simulink model "eDPWMv20matlab2020a"  (R2020a)
settings: Solver=VariableStepAuto  StartTime=0.0  StopTime=Tsim  MaxStep=MaxStep  RelTol=1e-3
values from neighbouring files (symbols this model uses):
  a = 1    [main.m]
  b = 1    [main.m]
  Default_NH = 1    [main.m]
  Default_NL = 0    [main.m]
  fs = 100e3    (= 100000)    [main.m]
  M = 0.3    [main.m]
  MaxStep = Ts/600    (= 1.66666666667e-08)    [main.m]
  PgnH = 1/20    (= 0.05)    [main.m]
  PgnL = 1/2    (= 0.5)    [main.m]
  Ts = 1/fs    (= 1e-05)    [main.m]
  Tsample = 1/fsample    (= 5e-06)    [main.m]
  Tsim = 8000*Ts    (= 0.08)    [main.m]
libraries: dspsigops x3
settings Model: Creator=pel  LastModifiedBy=Giovanni
settings DebuggingCC: UnconnectedInputMsg=none  UnconnectedOutputMsg=none  UnconnectedLineMsg=none
settings ModelReferenceCC: EnableRefExpFcnMdlSchedulingChecks=off
settings RTWCC: Description=Generic Real-Time Target  RTWVerbose=off

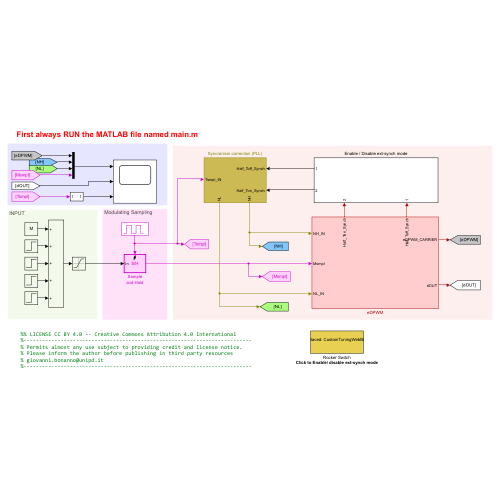
[thumbnail: Simulink's stored preview of the top-level diagram]
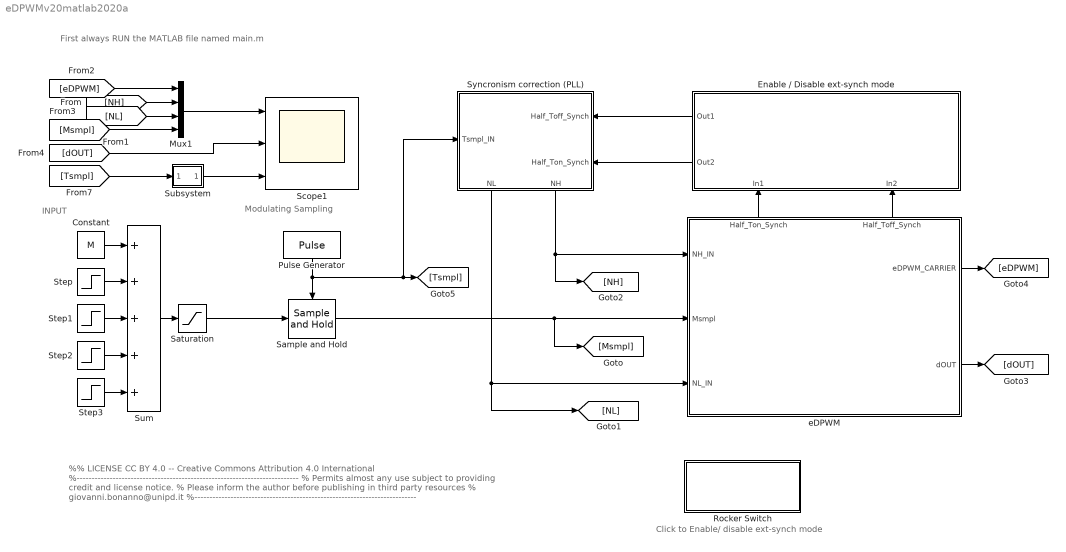
== system eDPWMv20matlab2020a ==
  note: First always RUN the MATLAB file named main.m
  note: Click to Enable/ disable ext-synch mode
  note: %% LICENSE CC BY 4.0 -- Creative Commons Attribution 4.0 International
      | %--------------------------------------------------------------------------
      | % Permits almost any use subject to providing credit and license notice.
      | % Please inform the author before publishing in third party resources
      | % giovanni.bonanno@unipd.it
      | %--------------------------------------------------------------------------
  note: Modulating Sampling
  note: INPUT
  Constant : Constant  Value=M  SampleTime=MaxStep
  Enable / Disable ext-synch mode : Subsystem
      settings: PortSchema="{\"entries\":[{\"content\":{\"sides\":[{\"content\":{},\"type\":\"ConnectorPlacement.EquallySpacedRectSide\",\"uuid\":\"202ee470-7674-402d-b318-20dd7def3ef2\"},{\"content\":{\"connectorIds\":[\"Out1\",\"Out2\"],\"side\":\"RIGHT\"},\"type\":\"ConnectorPlacement.EquallySpacedRectSide\",\"uuid\":\"6d0846ec-2558-4ef4-8253-932ba88cb3e0\"},{\"content\":{\"side\":\"TOP\"},\"type\":\"ConnectorPlacement.EquallySpacedRectSide\",\"uuid\":\"6d21b35b-35b5-4f81-8190-ca95fc47349c\"},{\"content\":{\"connectorIds\":[\"In1\",\"In2\"],\"side\":\"BOTTOM\"},\"type\":\"ConnectorPlacement.EquallySpacedRectSide\",\"uuid\":\"7a5dac1a-5bab-41fb-a369-e6d9d4d78f57\"}]},\"type\":\"ConnectorPlacement.EquallySpacedConnector\",\"uuid\":\"1e7bac81-8cd1-438e-9b37-227f8a4a31bc\"}],\"packageUris\":[\"http://schema.mathworks.com/mf0/Connector/R2020b\"],\"version\":\"1.0\"}"
  Mux1 : Mux
  Pulse Generator : DiscretePulseGenerator  PulseType=Time based  Period=Tsample  PulseWidth=50
  Rocker Switch : Subsystem  Description=Replaced Block  mask(Replaced Block){}
      mask help: This block has been replaced with an empty subsystem because it used functionality that is unavailable in Simulink R2020a.
      mask Display: fprintf('Replaced: %s\n','CustomTuningWebBlock')
  Sample and Hold : dspsigops/Sample and Hold  trig=Rising edge  initCond=M  latchinput=off
  Saturation : Saturate  UpperLimit=1  LowerLimit=0
  Scope1 : Scope  NumInputPorts=3
  Step : Step  Time=Ts*18-Ts/4  After=M/5  SampleTime=MaxStep
  Step1 : Step  Time=Ts*17+Ts/4  After=M/5  SampleTime=MaxStep
  Step2 : Step  Time=Tsim/18+Ts/4+Ts/2  After=M/20  SampleTime=MaxStep
  Step3 : Step  Time=Tsim/18+Ts/4+Ts  After=M/20  SampleTime=MaxStep
  Subsystem : Subsystem
  Sum : Sum  Inputs=+++++
  Syncronism correction (PLL) : Subsystem
      settings: PortSchema="{\"entries\":[{\"content\":{\"sides\":[{\"content\":{\"connectorIds\":[\"In1\"]},\"type\":\"ConnectorPlacement.EquallySpacedRectSide\",\"uuid\":\"af3382a3-5650-4608-9daa-49500a505952\"},{\"content\":{\"connectorIds\":[\"In2\",\"In3\"],\"side\":\"RIGHT\"},\"type\":\"ConnectorPlacement.EquallySpacedRectSide\",\"uuid\":\"51c7e400-8917-4fd6-8211-c90393d7470e\"},{\"content\":{\"side\":\"TOP\"},\"type\":\"ConnectorPlacement.EquallySpacedRectSide\",\"uuid\":\"30f0f9c1-e41e-4d95-bf06-70fe739465e7\"},{\"content\":{\"connectorIds\":[\"Out1\",\"Out2\"],\"side\":\"BOTTOM\"},\"type\":\"ConnectorPlacement.EquallySpacedRectSide\",\"uuid\":\"2c796cb0-67f8-4f41-8e4d-8aa9d4353e04\"}]},\"type\":\"ConnectorPlacement.EquallySpacedConnector\",\"uuid\":\"0b00b238-9597-4f72-adc3-115ce80e6692\"}],\"packageUris\":[\"http://schema.mathworks.com/mf0/Connector/R2020b\"],\"version\":\"1.0\"}"
  eDPWM : Subsystem
      settings: PortSchema="{\"entries\":[{\"content\":{\"sides\":[{\"content\":{\"connectorIds\":[\"In1\",\"In2\",\"In3\"]},\"type\":\"ConnectorPlacement.EquallySpacedRectSide\",\"uuid\":\"bf982af5-63e8-4a41-b560-11889742b778\"},{\"content\":{\"connectorIds\":[\"Out1\",\"Out2\"],\"side\":\"RIGHT\"},\"type\":\"ConnectorPlacement.EquallySpacedRectSide\",\"uuid\":\"a7efdfb9-974d-4c29-9fbc-b41dc0a107af\"},{\"content\":{\"connectorIds\":[\"Out3\",\"Out4\"],\"side\":\"TOP\"},\"type\":\"ConnectorPlacement.EquallySpacedRectSide\",\"uuid\":\"a9c88e29-f7b6-4c63-8087-8b423cce12c8\"},{\"content\":{\"side\":\"BOTTOM\"},\"type\":\"ConnectorPlacement.EquallySpacedRectSide\",\"uuid\":\"491d2149-b1e6-45d2-9cf1-74bcedeaf42d\"}]},\"type\":\"ConnectorPlacement.EquallySpacedConnector\",\"uuid\":\"8fa54b55-faee-4312-8aec-5ed5b37487a1\"}],\"packageUris\":[\"http://schema.mathworks.com/mf0/Connector/R2020b\"],\"version\":\"1.0\"}"
  wires:
  [NH] -> Mux1/2
  [eDPWM] -> Mux1/1
  [Msmpl] -> Mux1/4
  Saturation/1 -> Sample and Hold/1
  [NL] -> Mux1/3
  Mux1/1 -> Scope1/1
  [dOUT] -> Scope1/2
  Sum/1 -> Saturation/1
  Sample and Hold/1 -> eDPWM/2(Msmpl), [Msmpl]
  Pulse Generator/1 -> Sample and Hold/Trigger, Syncronism correction (PLL)/1(Tsmpl_IN), [Tsmpl]
  [Tsmpl] -> Subsystem/1(Inport)
  eDPWM/2(dOUT) -> [dOUT]
  Syncronism correction (PLL)/1(NL) -> eDPWM/3(NL_IN), [NL]
  Syncronism correction (PLL)/2(NH) -> eDPWM/1(NH_IN), [NH]
  eDPWM/1(eDPWM_CARRIER) -> [eDPWM]
  Subsystem/1(Out1) -> Scope1/3
  Constant/1 -> Sum/1
  Step/1 -> Sum/2
  Step1/1 -> Sum/3
  Step2/1 -> Sum/4
  Step3/1 -> Sum/5
  eDPWM/3(Half_Ton_Synch) -> Enable / Disable ext-synch mode/2(In1)
  eDPWM/4(Half_Toff_Synch) -> Enable / Disable ext-synch mode/1(In2)
  Enable / Disable ext-synch mode/1(Out1) -> Syncronism correction (PLL)/2(Half_Toff_Synch)
  Enable / Disable ext-synch mode/2(Out2) -> Syncronism correction (PLL)/3(Half_Ton_Synch)

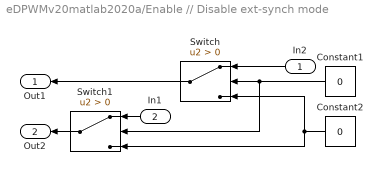
== system eDPWMv20matlab2020a/Enable // Disable ext-synch mode ==
  In2 : Inport
  In1 : Inport  Port=2
  Constant1 : Constant  Value=0
  Constant2 : Constant  Value=0
  Switch : Switch  Criteria=u2 > Threshold
  Switch1 : Switch  Criteria=u2 > Threshold
  Out1 : Outport
  Out2 : Outport  Port=2
  wires:
  In1/1 -> Switch1/1
  Constant2/1 -> Switch1/3, Switch/3
  In2/1 -> Switch/1
  Constant1/1 -> Switch1/2, Switch/2
  Switch1/1 -> Out2/1
  Switch/1 -> Out1/1

== system eDPWMv20matlab2020a/Rocker Switch ==

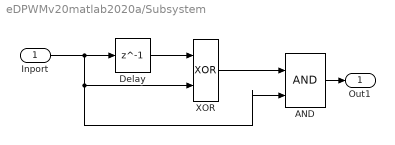
== system eDPWMv20matlab2020a/Subsystem ==
  Inport : Inport
  AND : Logic  IconShape=distinctive  AllPortsSameDT=off  OutDataTypeStr=boolean
  Delay : Delay  DelayLength=1  SampleTime=MaxStep
  XOR : Logic  Operator=XOR  IconShape=distinctive  AllPortsSameDT=off  OutDataTypeStr=boolean
  Out1 : Outport
  wires:
  Inport/1 -> AND/2, XOR/2, Delay/1
  Delay/1 -> XOR/1
  XOR/1 -> AND/1
  AND/1 -> Out1/1

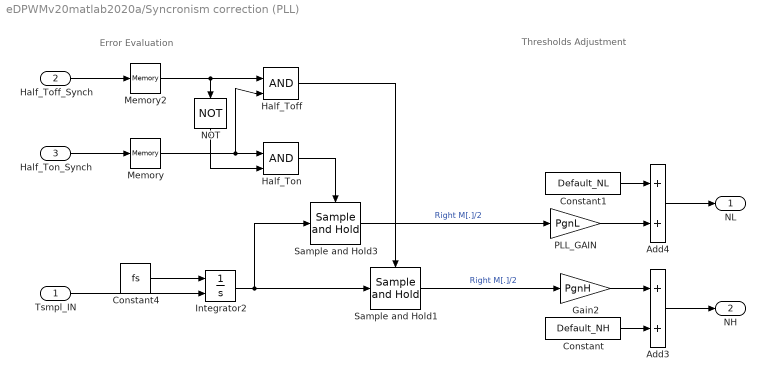
== system eDPWMv20matlab2020a/Syncronism correction (PLL) ==
  note: Thresholds Adjustment
  note: Error Evaluation
  Tsmpl_IN : Inport
  Half_Toff_Synch : Inport  Port=2
  Half_Ton_Synch : Inport  Port=3
  Add3 : Sum
  Add4 : Sum
  Constant : Constant  Value=Default_NH
  Constant1 : Constant  Value=Default_NL
  Constant4 : Constant  Value=fs
  Gain2 : Gain  Gain=PgnH
  Half_Toff : Logic  IconShape=distinctive  AllPortsSameDT=off  OutDataTypeStr=boolean
  Half_Ton : Logic  IconShape=distinctive  AllPortsSameDT=off  OutDataTypeStr=boolean
  Integrator2 : Integrator  ExternalReset=falling  InitialCondition=-0.25  UpperSaturationLimit=0.25  LowerSaturationLimit=-0.25
  Memory : Memory
  Memory2 : Memory
  NOT : Logic  Operator=NOT  IconShape=distinctive  AllPortsSameDT=off  OutDataTypeStr=boolean
  PLL_GAIN : Gain  Gain=PgnL
  Sample and Hold1 : dspsigops/Sample and Hold  trig=Rising edge  initCond=0  latchinput=off
  Sample and Hold3 : dspsigops/Sample and Hold  trig=Rising edge  initCond=0  latchinput=off
  NL : Outport
  NH : Outport  Port=2
  wires:
  Constant4/1 -> Integrator2/1
  Half_Ton/1 -> Sample and Hold3/Trigger
  Tsmpl_IN/1 -> Integrator2/2
  Half_Toff/1 -> Sample and Hold1/Trigger
  NOT/1 -> Half_Ton/2
  Half_Ton_Synch/1 -> Memory/1
  Constant1/1 -> Add4/1
  PLL_GAIN/1 -> Add4/2
  Constant/1 -> Add3/2
  Gain2/1 -> Add3/1
  Add4/1 -> NL/1
  Integrator2/1 -> Sample and Hold1/1, Sample and Hold3/1
  Add3/1 -> NH/1
  Sample and Hold1/1 -> Gain2/1  "Right M[.]/2"
  Sample and Hold3/1 -> PLL_GAIN/1  "Right M[.]/2"
  Memory2/1 -> NOT/1, Half_Toff/1
  Half_Toff_Synch/1 -> Memory2/1
  Memory/1 -> Half_Ton/1, Half_Toff/2

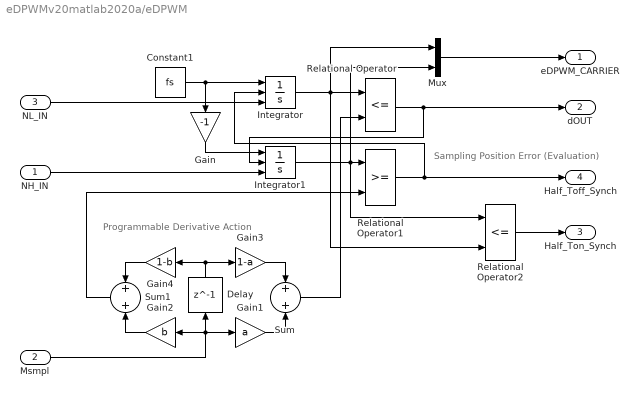
== system eDPWMv20matlab2020a/eDPWM ==
  note: Programmable Derivative Action
  note: Sampling Position Error (Evaluation)
  NH_IN : Inport
  Msmpl : Inport  Port=2
  NL_IN : Inport  Port=3
  Constant1 : Constant  Value=fs
  Delay : Delay  DelayLength=1  InitialCondition=0  SampleTime=Ts/2
  Gain : Gain  Gain=-1
  Gain1 : Gain  Gain=a
  Gain2 : Gain  Gain=b
  Gain3 : Gain  Gain=1-a
  Gain4 : Gain  Gain=1-b
  Integrator : Integrator  ExternalReset=falling  InitialConditionSource=external  InitialCondition=-0.15
  Integrator1 : Integrator  ExternalReset=falling  InitialConditionSource=external  InitialCondition=1
  Mux : Mux  Inputs=2
  Relational Operator : RelationalOperator  Operator=<=  OutDataTypeStr=boolean  RndMeth=Simplest
  Relational Operator1 : RelationalOperator  OutDataTypeStr=boolean  RndMeth=Simplest
  Relational Operator2 : RelationalOperator  Operator=<=  OutDataTypeStr=boolean  RndMeth=Simplest
  Sum : Sum
  Sum1 : Sum
  eDPWM_CARRIER : Outport
  dOUT : Outport  Port=2
  Half_Ton_Synch : Outport  Port=3
  Half_Toff_Synch : Outport  Port=4
  wires:
  Constant1/1 -> Integrator/1, Gain/1
  NL_IN/1 -> Integrator/3
  Integrator1/1 -> Mux/2, Relational Operator2/1, Relational Operator1/1
  Gain/1 -> Integrator1/1
  Relational Operator2/1 -> Half_Ton_Synch/1
  Integrator/1 -> Mux/1, Relational Operator2/2, Relational Operator/1
  Relational Operator1/1 -> Half_Toff_Synch/1, Integrator/2
  Relational Operator/1 -> Integrator1/2, dOUT/1
  Delay/1 -> Gain4/1, Gain3/1
  Gain3/1 -> Sum/1
  Sum/1 -> Relational Operator/2
  Sum1/1 -> Relational Operator1/2
  Gain1/1 -> Sum/2
  Msmpl/1 -> Gain2/1, Delay/1, Gain1/1
  Gain2/1 -> Sum1/2
  Gain4/1 -> Sum1/1
  NH_IN/1 -> Integrator1/3
  Mux/1 -> eDPWM_CARRIER/1
